simulink model "Single_Phase_Bridge_All_controlled"  (Simulink 7.5)
settings: Solver=ode15s  StartTime=0.0  StopTime=0.1  RelTol=1e-3
libraries: powerlib x8
settings Model: Creator=lm  LastModifiedBy=lm

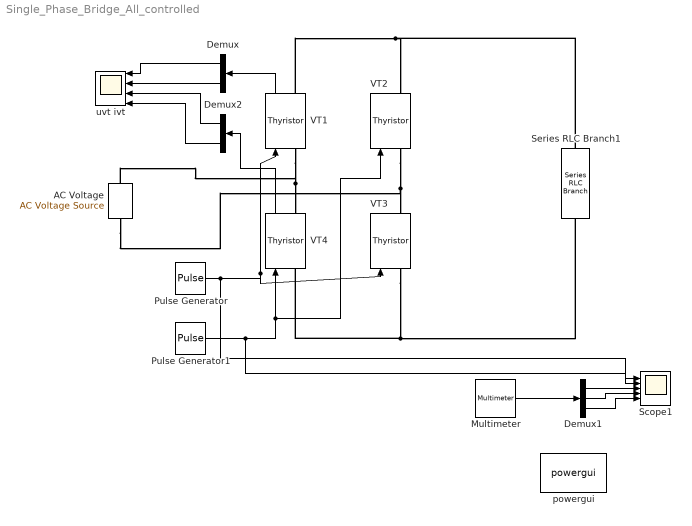
== system Single_Phase_Bridge_All_controlled ==
  AC Voltage : powerlib/Electrical Sources/AC Voltage Source  DialogController=POWERSYS.PowerSysDialog  SystemSampleTime=-1  Amplitude=220*sqrt(2)  Phase=0  Frequency=50  SampleTime=0  Measurements=Voltage
  Demux : Demux  Outputs=2
  Demux1 : Demux  Outputs=3
  Demux2 : Demux  Outputs=2
  Multimeter : powerlib/Measurements/Multimeter  SystemSampleTime=-1  PhasorSimulation=off  OutputType=Complex  sel=[2 1 3]  L=3  Gain=[1 1 1]  yselected={'Usrc: AC Voltage','Ub: Series RLC Branch1','Ib: Series RLC Branch1'};  PSBOutputType=1  PSBequivalent=0  AxesSetting=[0,0.1,-100,100]  Display=0  SavedBlockNames=-11
  Pulse Generator : DiscretePulseGenerator  PulseType=Time based  Amplitude=1  Period=0.02  PulseWidth=2.5  PhaseDelay=0.00333  SampleTime=1
  Pulse Generator1 : DiscretePulseGenerator  PulseType=Time based  Amplitude=1  Period=0.02  PulseWidth=2.5  PhaseDelay=0.01333  SampleTime=1
  Scope1 : Scope  NumInputPorts=5
      settings: YMin=-5~-5~-5~-5~-50  YMax=5~5~5~5~150  SaveName=ScopeData4
  Series RLC Branch1 : powerlib/Elements/Series RLC Branch  DialogController=POWERSYS.PowerSysDialog  PhysicalDomain=powersysdomain  SubClassName=unknown  LeftPortType=p1  RightPortType=p1  LConnTagsString=__new0  RConnTagsString=__new0  BranchType=RL  Resistance=2  Inductance=1e-2  SetiL0=off  InitialCurrent=0  Capacitance=1e-6  Setx0=off  InitialVoltage=0  Measurements=Branch voltage and current
  VT{1..4} (4 alike) : powerlib/Power Electronics/Thyristor  DialogController=POWERSYS.PowerSysDialog  SystemSampleTime=-1  Ron=0.001  Lon=0  Vf=0.8  IC=0  Rs=500  Cs=250e-9  Measurements=on
  powergui : powerlib/powergui  Priority=1  SystemSampleTime=-1  SimulationMode=Discrete  SampleTime=50e-6  frequency=60  SPID=off  DisableSnubberDevices=off  DisableRonSwitches=off  DisableVfSwitches=off  SwTol=0  Interpol=off  frequencyindice=50  echomessages=off  HookPort=off  DisplayEquations=off  FunctionMessages=off  EnableUseOfTLC=off  x0status=blocks  RestoreLinks=warning  ResistiveCurrentMeasurement=off  Ylog=off  Xlog=on  ShowGrid=off  save=off  variable=ZData  ZoomFFT=off  StartTime=0.0  cycles=1  DisplayStyle=1  FreqAxis=off  MaxFrequency=1000  frequencyindicesteady=1  display=off  methode=off
  uvt ivt : Scope  NumInputPorts=4
      settings: YMin=-5~-5~-5~-5  YMax=5~5~5~5
  wires:
  Pulse Generator/1 -> VT1/1, VT3/1, Scope1/1
  Pulse Generator1/1 -> VT4/1, VT2/1, Scope1/2
  VT1/1 -> Demux/1
  Demux/1 -> uvt ivt/1
  Demux/2 -> uvt ivt/2
  Multimeter/1 -> Demux1/1
  VT4/1 -> Demux2/1
  Demux2/1 -> uvt ivt/3
  Demux2/2 -> uvt ivt/4
  Demux1/1 -> Scope1/3
  Demux1/2 -> Scope1/4
  Demux1/3 -> Scope1/5
  connections:
  VT1/LConn1 -- VT4/RConn1 -- AC Voltage/RConn1
  Series RLC Branch1/RConn1 -- VT3/LConn1 -- VT4/LConn1
  Series RLC Branch1/LConn1 -- VT1/RConn1 -- VT2/RConn1
  AC Voltage/LConn1 -- VT2/LConn1 -- VT3/RConn1
